simulink model "reducedobserver_regulatorcontroller_firstpoles_s"  (R2021b)
settings: Solver=VariableStepAuto  StartTime=0.0  StopTime=15  RelTol=1e-3
undefined symbols (not defined in the file): A_1, A_2, Ao, B_1, Bo, Co, K1, L_reduced1, Q1, Q2
settings Model: Creator=nima8  LastModifiedBy=nima8

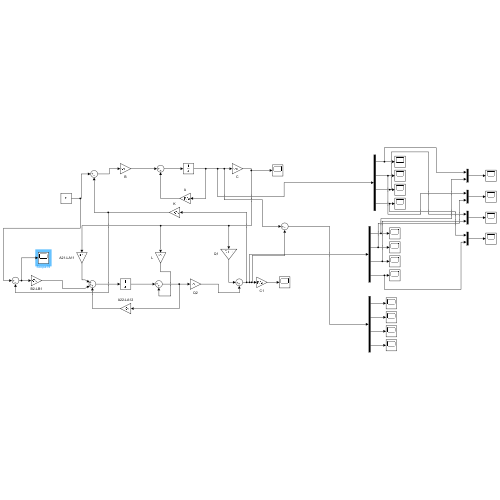
[thumbnail: Simulink's stored preview of the top-level diagram]
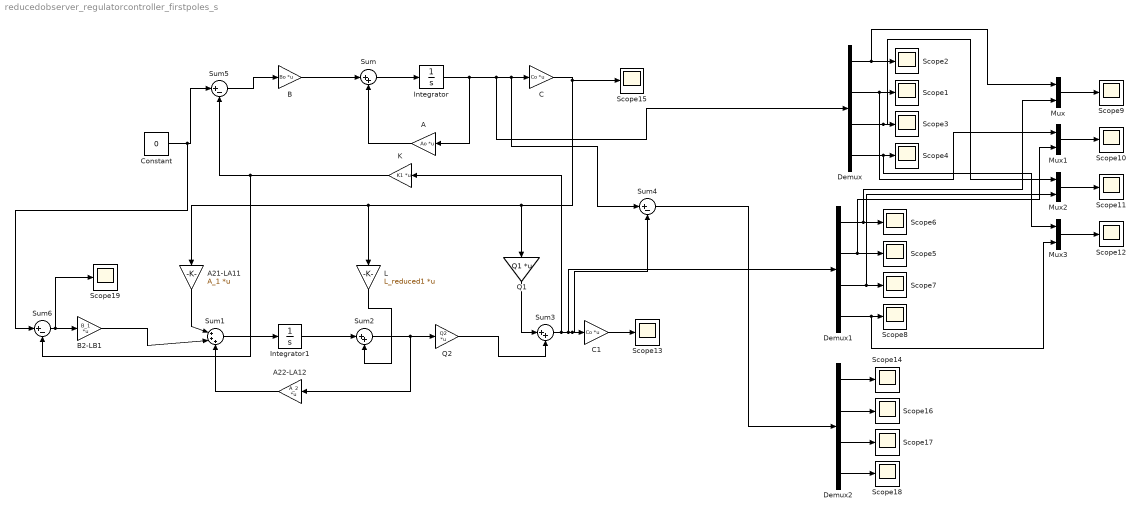
== system reducedobserver_regulatorcontroller_firstpoles_s ==
  A : Gain  Gain=Ao  Multiplication=Matrix(K*u)
  A21-LA11 : Gain  Gain=A_1  Multiplication=Matrix(K*u)
  A22-LA12 : Gain  Gain=A_2  Multiplication=Matrix(K*u)
  B : Gain  Gain=Bo  Multiplication=Matrix(K*u)
  B2-LB1 : Gain  Gain=B_1  Multiplication=Matrix(K*u)
  C : Gain  Gain=Co  Multiplication=Matrix(K*u)
  C1 : Gain  Gain=Co  Multiplication=Matrix(K*u)
  Constant : Constant  Value=0
  Demux : Demux
  Demux1 : Demux
  Demux2 : Demux
  Integrator : Integrator  InitialCondition=[1 0.5 -1 2]
  Integrator1 : Integrator  InitialCondition=[-2 3 -2]
  K : Gain  Gain=K1  Multiplication=Matrix(K*u)
  L : Gain  Gain=L_reduced1  Multiplication=Matrix(K*u)
  Mux{,1..3} (4 alike) : Mux  Inputs=2
  Q1 : Gain  Gain=Q1  Multiplication=Matrix(K*u)
  Q2 : Gain  Gain=Q2  Multiplication=Matrix(K*u)
  Scope{1..19} (19 alike) : Scope
  Sum : Sum  Inputs=|++
  Sum1 : Sum  Inputs=|+++
  Sum2 : Sum  Inputs=|++
  Sum3 : Sum  Inputs=|++
  Sum4 : Sum  Inputs=|+-
  Sum5 : Sum  Inputs=|+-
  Sum6 : Sum  Inputs=|+-
  wires:
  Demux1/1 -> Mux/2, Scope6/1
  Demux1/3 -> Mux2/2, Scope7/1
  Demux/1 -> Mux/1, Scope2/1
  Mux2/1 -> Scope11/1
  Integrator1/1 -> Sum2/1
  Sum/1 -> Integrator/1
  A22-LA12/1 -> Sum1/3
  Q1/1 -> Sum3/1
  B/1 -> Sum/1
  Demux/4 -> Mux3/1, Scope4/1
  A/1 -> Sum/2
  C/1 -> Scope15/1, A21-LA11/1, L/1, Q1/1
  Demux/3 -> Mux2/1, Scope3/1
  Mux1/1 -> Scope10/1
  Sum1/1 -> Integrator1/1
  Q2/1 -> Sum3/2
  A21-LA11/1 -> Sum1/1
  Demux2/3 -> Scope17/1
  Mux3/1 -> Scope12/1
  B2-LB1/1 -> Sum1/2
  Demux1/4 -> Mux3/2, Scope8/1
  Integrator/1 -> Demux/1, Sum4/1, C/1, A/1
  Sum3/1 -> K/1, Demux1/1, Sum4/2, C1/1
  C1/1 -> Scope13/1
  Mux/1 -> Scope9/1
  Sum4/1 -> Demux2/1
  Demux2/4 -> Scope18/1
  Demux/2 -> Mux1/1, Scope1/1
  Sum2/1 -> A22-LA12/1, Q2/1
  Demux1/2 -> Mux1/2, Scope5/1
  Demux2/2 -> Scope16/1
  Demux2/1 -> Scope14/1
  L/1 -> Sum2/2
  Constant/1 -> Sum6/1, Sum5/1
  Sum5/1 -> B/1
  K/1 -> Sum6/2, Sum5/2
  Sum6/1 -> Scope19/1, B2-LB1/1
